simulink model "shell_eco_mainV8c"  (R2023b)
settings: Solver=ode23tb  StartTime=0.0  StopTime=t_end  MaxStep=0.1  RelTol=1e-3
undefined symbols (not defined in the file): A, Cd, Crr, effic_drive, effic_engine, EngineRPM_map, EngineTorque_map, g, G, LHV, m, r_w, rho, RPM_idle, RPM_max, v0, v_high_on, v_low_on, x0
settings Model: Creator=canfi  LastModifiedBy=canfi
settings SolverCC: MaxConsecutiveZCs=10000  ZeroCrossAlgorithm=Adaptive
settings DebuggingCC: IgnoredZcDiagnostic=none

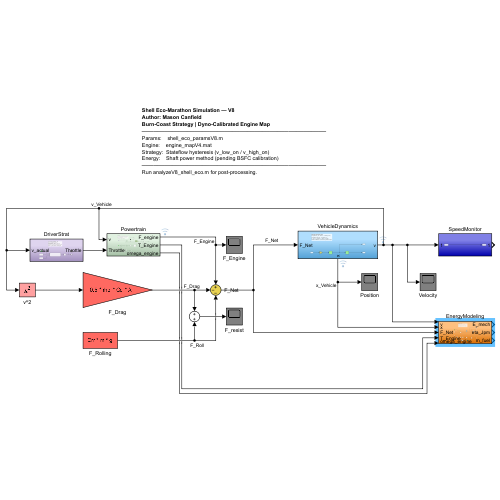
[thumbnail: Simulink's stored preview of the top-level diagram]
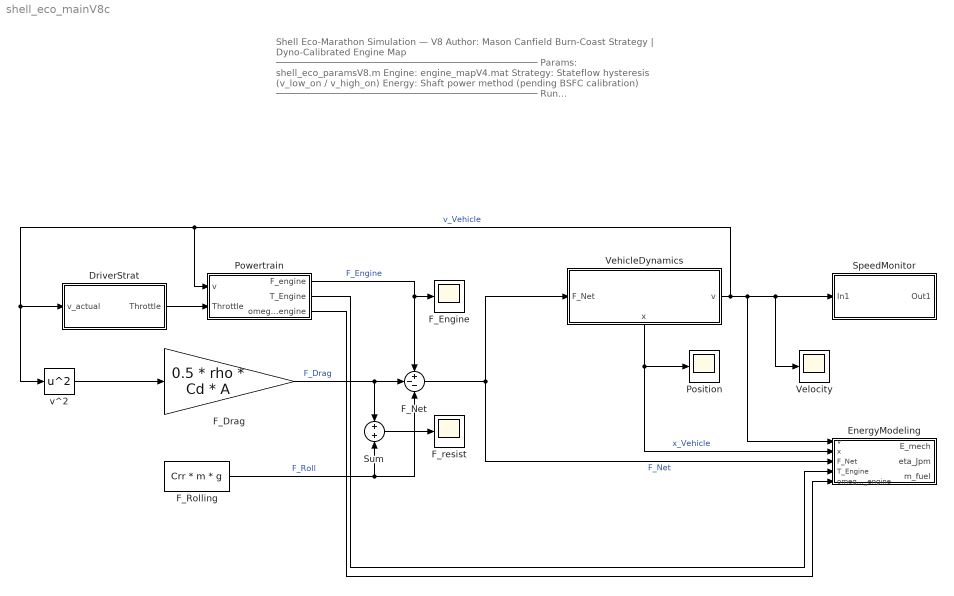
== system shell_eco_mainV8c ==
  note: Shell Eco-Marathon Simulation — V8
      | Author: Mason Canfield
      | Burn-Coast Strategy | Dyno-Calibrated Engine Map
      | ─────────────────────────────────────────────────
      | Params: shell_eco_paramsV8.m
      | Engine: engine_mapV4.mat
      | Strategy: Stateflow hysteresis (v_low_on / v_high_on)
      | Energy: Shaft power method (pending BSFC calibration)
      | ─────────────────────────────────────────────────
      | Run analyzeV8_shell_eco.m for post-processing.
  DriverStrat : Subsystem
  EnergyModeling : Subsystem
  F_Drag : Gain  Gain=0.5 * rho * Cd * A
  F_Engine : Scope
  F_Net : Sum  Inputs=+--
  F_Rolling : Constant  Value=Crr * m * g
  F_resist : Scope
  Position : Scope
  Powertrain : Subsystem
  SpeedMonitor : Subsystem
  Sum : Sum
  VehicleDynamics : Subsystem
      settings: PortSchema="{\"entries\":[{\"content\":{\"sides\":[{\"content\":{\"connectorIds\":[\"In1\"]},\"type\":\"ConnectorPlacement.EquallySpacedRectSide\",\"uuid\":\"dfdfb956-2909-41e2-ad74-eec43401073f\"},{\"content\":{\"connectorIds\":[\"Out1\"],\"side\":\"RIGHT\"},\"type\":\"ConnectorPlacement.EquallySpacedRectSide\",\"uuid\":\"11842bdc-6931-40ed-a403-b6947f0a89a0\"},{\"content\":{\"side\":\"TOP\"},\"type\":\"ConnectorPlacement.EquallySpacedRectSide\",\"uuid\":\"79a25e54-4e3e-453f-b478-21948a5fad51\"},{\"content\":{\"connectorIds\":[\"Out2\"],\"side\":\"BOTTOM\"},\"type\":\"ConnectorPlacement.EquallySpacedRectSide\",\"uuid\":\"b1ef2620-ee40-4a96-8fe4-d7ac3411631d\"}]},\"type\":\"ConnectorPlacement.EquallySpacedConnector\",\"uuid\":\"a04151ff-9342-40bb-a5c2-12dc5cb0586b\"}],\"packageUris\":[\"http://schema.mathworks.com/mf0/Connector/R2020b\"],\"version\":\"1.0\"}"
  Velocity : Scope
  v^2 : Math  Operator=square
  wires:
  DriverStrat/1(Throttle) -> Powertrain/2(Throttle)
  VehicleDynamics/2(x) -> EnergyModeling/2(x), Position/1  "x_Vehicle"
  VehicleDynamics/1(v) -> SpeedMonitor/1(In1), Velocity/1, EnergyModeling/1(v), Powertrain/1(v), v^2/1, DriverStrat/1(v_actual)  "v_Vehicle"
  Powertrain/1(F_engine) -> F_Engine/1, F_Net/1  "F_Engine"
  v^2/1 -> F_Drag/1
  F_Net/1 -> EnergyModeling/3(F_Net), VehicleDynamics/1(F_Net)  "F_Net"
  F_Rolling/1 -> F_Net/3, Sum/2  "F_Roll"
  F_Drag/1 -> F_Net/2, Sum/1  "F_Drag"
  Sum/1 -> F_resist/1
  Powertrain/2(T_Engine) -> EnergyModeling/4(T_Engine)
  Powertrain/3(omega_engine) -> EnergyModeling/5(omega_engine)

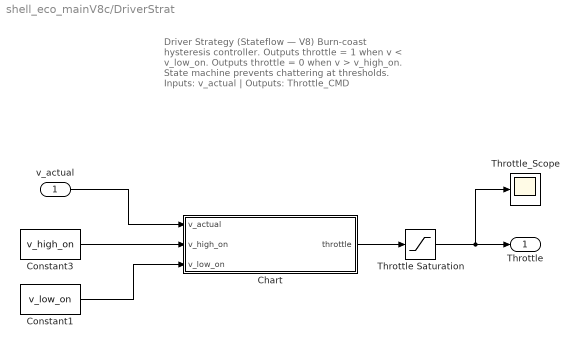
== system shell_eco_mainV8c/DriverStrat ==
  note: Driver Strategy (Stateflow — V8)
      | Burn-coast hysteresis controller.
      | Outputs throttle = 1 when v < v_low_on.
      | Outputs throttle = 0 when v > v_high_on.
      | State machine prevents chattering at thresholds.
      | Inputs: v_actual | Outputs: Throttle_CMD
  v_actual : Inport
  Chart : Stateflow chart  TreatAsAtomicUnit=on  SystemSampleTime=0.1
  Constant1 : Constant  Value=v_low_on
  Constant3 : Constant  Value=v_high_on
  Throttle Saturation : Saturate  UpperLimit=1  LowerLimit=0
  Throttle_Scope : Scope
  Throttle : Outport
  wires:
  v_actual/1 -> Chart/1(v_actual)
  Constant1/1 -> Chart/3(v_low_on)
  Constant3/1 -> Chart/2(v_high_on)
  Chart/1(throttle) -> Throttle Saturation/1
  Throttle Saturation/1 -> Throttle_Scope/1, Throttle/1

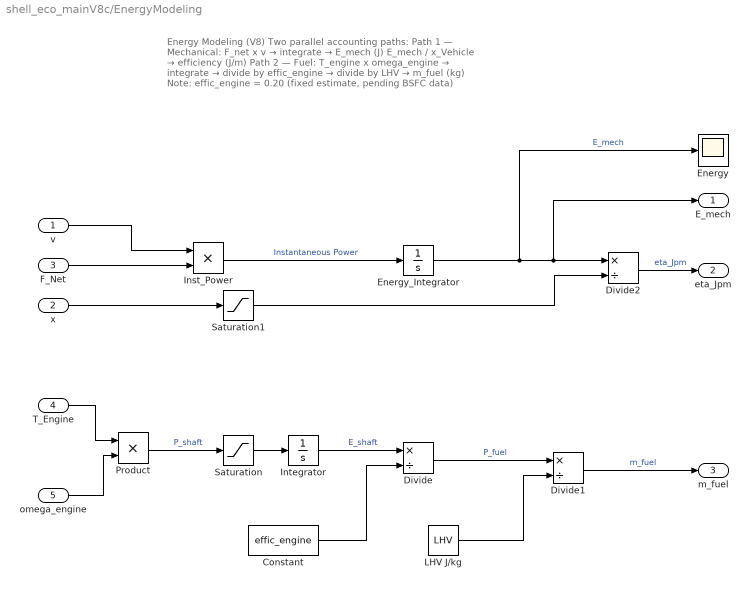
== system shell_eco_mainV8c/EnergyModeling ==
  note: Energy Modeling (V8)
      | Two parallel accounting paths:
      | Path 1 — Mechanical: F_net x v → integrate → E_mech (J)
      | E_mech / x_Vehicle → efficiency (J/m)
      | Path 2 — Fuel: T_engine x omega_engine → integrate
      | → divide by effic_engine → divide by LHV
      | → m_fuel (kg)
      | Note: effic_engine = 0.20 (fixed estimate, pending BSFC data)
  v : Inport
  x : Inport  Port=2
  F_Net : Inport  Port=3
  T_Engine : Inport  Port=4
  omega_engine : Inport  Port=5
  Constant : Constant  Value=effic_engine
  Divide : Product  Inputs=*/
  Divide1 : Product  Inputs=*/
  Divide2 : Product  Inputs=*/
  Energy : Scope
  Energy_Integrator : Integrator
  Inst_Power : Product
  Integrator : Integrator
  LHV J/kg : Constant  Value=LHV
  Product : Product
  Saturation : Saturate  UpperLimit=inf  LowerLimit=0
  Saturation1 : Saturate  UpperLimit=inf  LowerLimit=0.001
  E_mech : Outport
  eta_Jpm : Outport  Port=2
  m_fuel : Outport  Port=3
  wires:
  v/1 -> Inst_Power/1
  F_Net/1 -> Inst_Power/2
  Inst_Power/1 -> Energy_Integrator/1  "Instantaneous Power"
  Energy_Integrator/1 -> E_mech/1, Divide2/1, Energy/1  "E_mech"
  LHV J/kg/1 -> Divide1/2
  Divide1/1 -> m_fuel/1  "m_fuel"
  T_Engine/1 -> Product/1
  omega_engine/1 -> Product/2
  Product/1 -> Saturation/1  "P_shaft"
  Constant/1 -> Divide/2
  Divide/1 -> Divide1/1  "P_fuel"
  Integrator/1 -> Divide/1  "E_shaft"
  Divide2/1 -> eta_Jpm/1  "eta_Jpm"
  Saturation/1 -> Integrator/1
  x/1 -> Saturation1/1
  Saturation1/1 -> Divide2/2

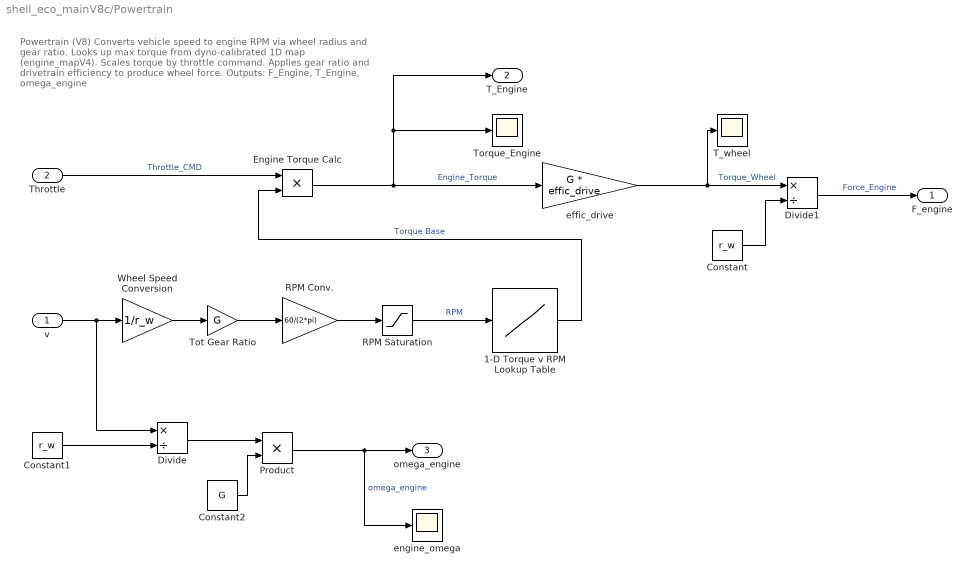
== system shell_eco_mainV8c/Powertrain ==
  note: Powertrain (V8)
      | Converts vehicle speed to engine RPM via wheel radius and gear ratio.
      | Looks up max torque from dyno-calibrated 1D map (engine_mapV4).
      | Scales torque by throttle command.
      | Applies gear ratio and drivetrain efficiency to produce wheel force.
      | Outputs: F_Engine, T_Engine, omega_engine
  v : Inport
  Throttle : Inport  Port=2
  1-D Torque v RPM Lookup Table : Lookup_n-D  NumberOfTableDimensions=1  BreakpointsForDimension1=EngineRPM_map  Table=EngineTorque_map  ExtrapMethod=Clip  InternalRulePriority=Speed  RndMeth=Simplest
  Constant : Constant  Value=r_w
  Constant1 : Constant  Value=r_w
  Constant2 : Constant  Value=G
  Divide : Product  Inputs=*/
  Divide1 : Product  Inputs=*/
  Engine Torque Calc : Product
  Product : Product
  RPM Conv. : Gain  Gain=60/(2*pi)
  RPM Saturation : Saturate  UpperLimit=RPM_max  LowerLimit=RPM_idle
  T_wheel : Scope
  Torque_Engine : Scope
  Tot Gear Ratio : Gain  Gain=G
  Wheel Speed Conversion : Gain  Gain=1/r_w
  effic_drive : Gain  Gain=G * effic_drive
  engine_omega : Scope
  F_engine : Outport
  T_Engine : Outport  Port=2
  omega_engine : Outport  Port=3
  wires:
  Wheel Speed Conversion/1 -> Tot Gear Ratio/1
  Tot Gear Ratio/1 -> RPM Conv./1
  v/1 -> Divide/1, Wheel Speed Conversion/1
  RPM Conv./1 -> RPM Saturation/1
  1-D Torque v RPM Lookup Table/1 -> Engine Torque Calc/2  "Torque Base"
  Throttle/1 -> Engine Torque Calc/1  "Throttle_CMD"
  Engine Torque Calc/1 -> T_Engine/1, Torque_Engine/1, effic_drive/1  "Engine_Torque"
  Divide1/1 -> F_engine/1  "Force_Engine"
  RPM Saturation/1 -> 1-D Torque v RPM Lookup Table/1  "RPM"
  effic_drive/1 -> T_wheel/1, Divide1/1  "Torque_Wheel"
  Constant/1 -> Divide1/2
  Constant1/1 -> Divide/2
  Divide/1 -> Product/1
  Constant2/1 -> Product/2
  Product/1 -> engine_omega/1, omega_engine/1  "omega_engine"

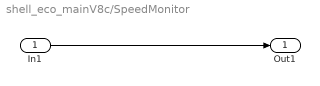
== system shell_eco_mainV8c/SpeedMonitor ==
  In1 : Inport
  Out1 : Outport
  wires:
  In1/1 -> Out1/1

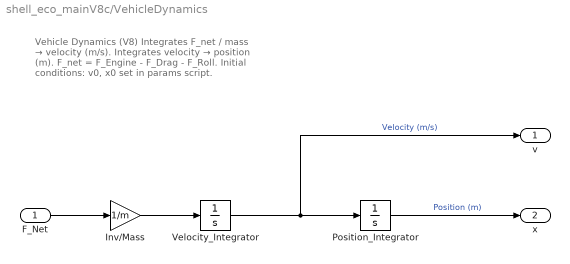
== system shell_eco_mainV8c/VehicleDynamics ==
  note: Vehicle Dynamics (V8)
      | Integrates F_net / mass → velocity (m/s).
      | Integrates velocity → position (m).
      | F_net = F_Engine - F_Drag - F_Roll.
      | Initial conditions: v0, x0 set in params script.
  F_Net : Inport
  Inv/Mass : Gain  Gain=1/m
  Position_Integrator : Integrator  InitialCondition=x0
  Velocity_Integrator : Integrator  InitialCondition=v0
  v : Outport
  x : Outport  Port=2
  wires:
  Inv/Mass/1 -> Velocity_Integrator/1
  Velocity_Integrator/1 -> v/1, Position_Integrator/1  "Velocity (m/s)"
  Position_Integrator/1 -> x/1  "Position (m)"
  F_Net/1 -> Inv/Mass/1

== stateflow chart shell_eco_mainV8c/DriverStrat/Chart ==
  settings: updateMethod=DISCRETE  sampleTime=0.1
  state BURN
    entry: throttle = 1;
  state COAST
    entry: throttle = 0;
  (default) -> BURN
  BURN -> COAST : [v_actual >= v_high_on]
  COAST -> BURN : [v_actual <= v_low_on]
  data: v_actual input; v_high_on input; v_low_on input; throttle output
